simulink model "test"  (R2015a)
settings: Solver=ode45  StartTime=0.0  StopTime=10.0  RelTol=1e-3
libraries: simulink x1
settings Model: Creator=ANSYSVLAD  LastModifiedBy=ANSYSVLAD

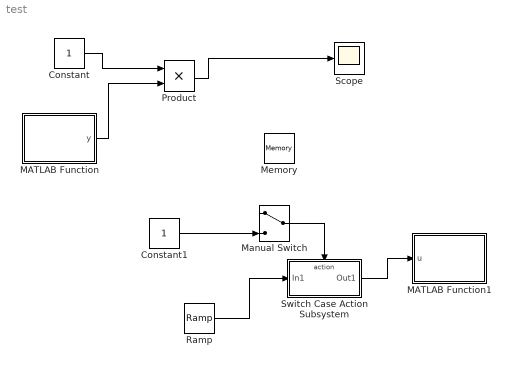
== system test ==
  Constant : Constant
  Constant1 : Constant
  MATLAB Function : MATLAB Function  TreatAsAtomicUnit=on
  MATLAB Function1 : MATLAB Function  TreatAsAtomicUnit=on
  Manual Switch : ManualSwitch
  Memory : Memory
  Product : Product
  Ramp : simulink/Sources/Ramp  slope=1  start=0  X0=0
  Scope : Scope
  Switch Case Action Subsystem : Subsystem  TreatAsAtomicUnit=on
  wires:
  Constant/1 -> Product/1
  Product/1 -> Scope/1
  MATLAB Function/1(y) -> Product/2
  Ramp/1 -> Switch Case Action Subsystem/1(In1)
  Switch Case Action Subsystem/1(Out1) -> MATLAB Function1/1(u)
  Manual Switch/1 -> Switch Case Action Subsystem/Action
  Constant1/1 -> Manual Switch/2

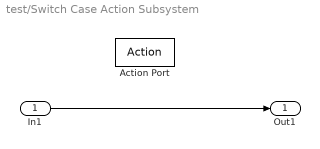
== system test/Switch Case Action Subsystem ==
  In1 : Inport
  Action Port : ActionPort
  Out1 : Outport
  wires:
  In1/1 -> Out1/1

== matlab function test/MATLAB Function1 ==
  data: u input
function fcn2(u)
%#codegen

test = u;

== matlab function test/MATLAB Function ==
  data: y output
function y = fcn()
%#codegen

y = test;
